simulink model "DataAcquisition_SimplePendulum"  (R2015b)
settings: Solver=VariableStepAuto  StartTime=0.0  StopTime=710  RelTol=1e-3
InitFcn:
  | T=0.005;
StopFcn:
  | % save file to results folder
  | name = datestr(now);
  | name = strrep(name,' ','_');
  | name = strrep(name,':','-');
  | 
  | name = strcat('out_sw_inn_fw_ramps_',name);
  | save(name)
  | 
  | 
  | % out_sw_inn_bw_10_
  | % out_sw_inn_fw_10_
  | 
  | % out_sw_inn_0fw_ramp_
  | % out_sw_inn_9fw_ramp_
  | % out_sw_inn_28d21fw_ramp_1
  | 
  | % inn_sw_out_fw_10_
  | % inn_sw_out_bw_10_
  | 
  | % fall_fw_
undefined symbols (not defined in the file or in its folder): National_Instruments, PCI
libraries: sldrtlib x3, simulink x2
settings Model: Creator=mounir  LastModifiedBy=mounir

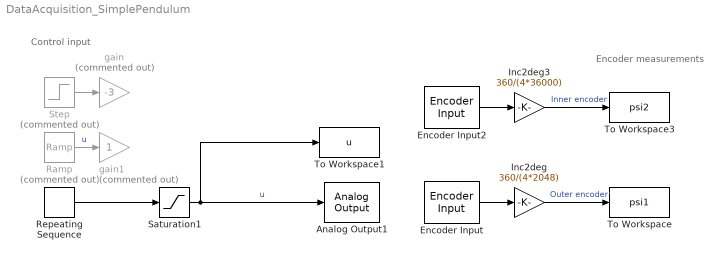
== system DataAcquisition_SimplePendulum ==
  note: Encoder
      | measurements
  note: Control input
  Analog Output1 : sldrtlib/Analog Output  SampleTime=T  MaxMissedTicks=Inf  ShowMissedTicks=off  YieldWhenWaiting=off  DrvName=National_Instruments/PCI-6221  DrvAddress=4294967295  DrvOptions=[0 0 0 2 2]  Channels=1  RangeMode=1  VoltRange=1  InitialValue=0  FinalValue=0
      settings: AttributesFormatString=National Instruments\nPCI-6221 [auto]
  Encoder Input : sldrtlib/Encoder Input  SampleTime=T  MaxMissedTicks=Inf  ShowMissedTicks=off  YieldWhenWaiting=off  DrvName=National_Instruments/PCI-6221  DrvAddress=4294967295  DrvOptions=[0 0 0 2 2]  Channels=1  QuadMode=3  IndexPulse=2  InputFilter=Inf  DataType=1
      settings: AttributesFormatString=National Instruments\nPCI-6221 [auto]
  Encoder Input2 : sldrtlib/Encoder Input  SampleTime=T  MaxMissedTicks=Inf  ShowMissedTicks=off  YieldWhenWaiting=off  DrvName=National_Instruments/PCI-6221  DrvAddress=4294967295  DrvOptions=[0 0 0 2 2]  Channels=2  QuadMode=3  IndexPulse=2  InputFilter=Inf  DataType=1
      settings: AttributesFormatString=National Instruments\nPCI-6221 [auto]
  Inc2deg : Gain  Gain=360/(4*2048)
  Inc2deg3 : Gain  Gain=360/(4*36000)
  Ramp : simulink/Sources/Ramp  Commented=on  slope=0.2  start=0  X0=0
  Repeating Sequence : simulink/Sources/Repeating Sequence  rep_seq_t=[0 10 65 70]  rep_seq_y=[0 0 10 10]
  Saturation1 : Saturate  UpperLimit=10  LowerLimit=-10
  Step : Step  Commented=on  SampleTime=0
  To Workspace : ToWorkspace  VariableName=psi1  SaveFormat=Timeseries  SampleTime=T
  To Workspace1 : ToWorkspace  VariableName=u  SaveFormat=Timeseries  SampleTime=T
  To Workspace3 : ToWorkspace  VariableName=psi2  SaveFormat=Timeseries  SampleTime=T
  gain : Gain  Commented=on  Gain=-3
  gain1 : Gain  Commented=on
  wires:
  Encoder Input/1 -> Inc2deg/1
  Ramp/1 -> gain1/1  "u"
  Inc2deg/1 -> To Workspace/1  "Outer encoder"
  Repeating Sequence/1 -> Saturation1/1
  Saturation1/1 -> To Workspace1/1, Analog Output1/1  "u"
  Encoder Input2/1 -> Inc2deg3/1
  Inc2deg3/1 -> To Workspace3/1  "Inner encoder"
  Step/1 -> gain/1
